simulink subsystem "Battery"  (R2022a)
settings: Solver=VariableStepAuto  StartTime=0.0  StopTime=10.0  RelTol=1e-3
settings Model: Creator=mateu  LastModifiedBy=mateu

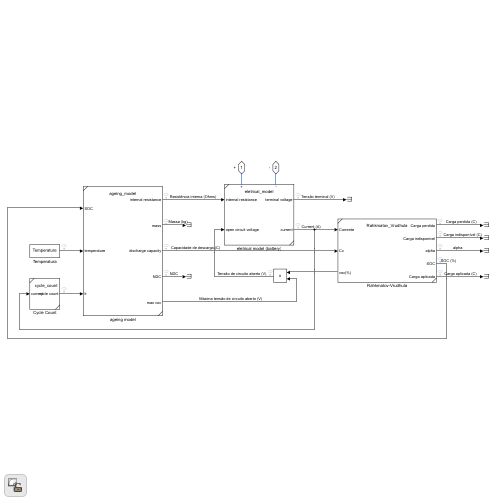
[thumbnail: Simulink's stored preview of the top-level diagram]
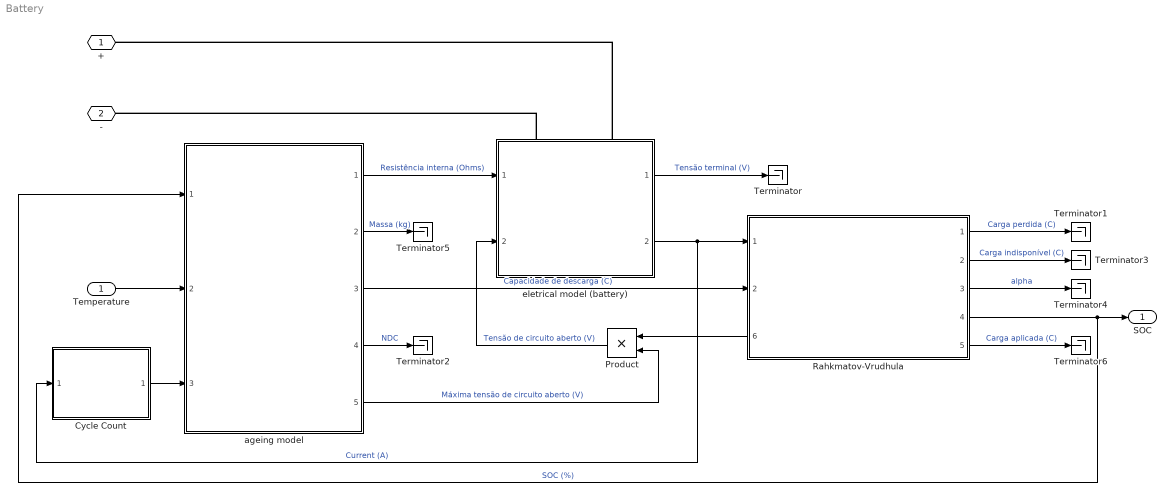
== system Battery ==
  Temperature : Inport
  Cycle Count : Subsystem  ReferencedSubsystem=cycle_count
  Product : Product
  Rahkmatov-Vrudhula : Subsystem  ReferencedSubsystem=Rahkmatov_Vrudhula
      settings: PortSchema="{\"entries\":[{\"content\":{\"sides\":[{\"content\":{\"connectorIds\":[\"In1\",\"In2\",\"Out6\"]},\"type\":\"ConnectorPlacement.EquallySpacedRectSide\",\"uuid\":\"83f3e873-db9f-47d1-b7c3-7eda48a10b32\"},{\"content\":{\"connectorIds\":[\"Out1\",\"Out2\",\"Out3\",\"Out4\",\"Out5\"],\"side\":\"RIGHT\"},\"type\":\"ConnectorPlacement.EquallySpacedRectSide\",\"uuid\":\"48ac6012-cdb4-4752-bc48-afa50bea9f0a\"},{\"content\":{\"connectorIds\":[],\"side\":\"TOP\"},\"type\":\"ConnectorPlacement.EquallySpacedRectSide\",\"uuid\":\"9cdc78bf-a718-48f1-92e6-e4070151caee\"}]},\"type\":\"ConnectorPlacement.EquallySpacedConnector\",\"uuid\":\"a231f58d-8e16-4cb4-bc80-61541bcf90eb\"}],\"packageUris\":[\"http://schema.mathworks.com/mf0/Connector/R2020b\"],\"version\":\"1.0\"}"
  Terminator{,1..6} (7 alike) : Terminator
  ageing model : Subsystem  ReferencedSubsystem=ageing_model
  eletrical model (battery) : Subsystem  ReferencedSubsystem=eletrical_model
      settings: PortSchema="{\"entries\":[{\"content\":{\"sides\":[{\"content\":{\"connectorIds\":[\"In1\",\"In2\"]},\"type\":\"ConnectorPlacement.EquallySpacedRectSide\",\"uuid\":\"e6309cc0-43d6-42db-b46d-fb5b38de698a\"},{\"content\":{\"connectorIds\":[\"Out1\",\"Out2\"],\"side\":\"RIGHT\"},\"type\":\"ConnectorPlacement.EquallySpacedRectSide\",\"uuid\":\"a3175445-87c0-47b1-a387-288225673634\"},{\"content\":{\"connectorIds\":[\"LConn2\",\"LConn1\"],\"side\":\"TOP\"},\"type\":\"ConnectorPlacement.EquallySpacedRectSide\",\"uuid\":\"f4aa44c9-f4dc-4aa8-a833-4f30710d8785\"},{\"content\":{\"connectorIds\":[],\"side\":\"BOTTOM\"},\"type\":\"ConnectorPlacement.EquallySpacedRectSide\",\"uuid\":\"f1117e0f-3189-4255-ad3f-4e2c31bb9482\"}]},\"type\":\"ConnectorPlacement.EquallySpacedConnector\",\"uuid\":\"e93a8d23-5e48-4dda-985c-f45f4ee27765\"}],\"packageUris\":[\"http://schema.mathworks.com/mf0/Connector/R2020b\"],\"version\":\"1.0\"}"
  + : PMIOPort  Side=Left
  - : PMIOPort  Port=2  Side=Left
  SOC : Outport
  wires:
  ageing model/2 -> Terminator5/1  "Massa (kg)"
  ageing model/4 -> Terminator2/1  "NDC"
  Temperature/1 -> ageing model/2
  ageing model/1 -> eletrical model (battery)/1  "Resistência interna (Ohms)"
  Cycle Count/1 -> ageing model/3
  eletrical model (battery)/2 -> Rahkmatov-Vrudhula/1, Cycle Count/1  "Current (A)"
  Rahkmatov-Vrudhula/4 -> ageing model/1, SOC/1  "SOC (%)"
  Rahkmatov-Vrudhula/3 -> Terminator4/1  "alpha"
  ageing model/5 -> Product/2  "Máxima tensão de circuito aberto (V)"
  Product/1 -> eletrical model (battery)/2  "Tensão de circuito aberto (V)"
  Rahkmatov-Vrudhula/5 -> Terminator6/1  "Carga aplicada (C)"
  eletrical model (battery)/1 -> Terminator/1  "Tensão terminal (V)"
  Rahkmatov-Vrudhula/2 -> Terminator3/1  "Carga indisponível (C)"
  Rahkmatov-Vrudhula/1 -> Terminator1/1  "Carga perdida (C)"
  Rahkmatov-Vrudhula/6 -> Product/1
  ageing model/3 -> Rahkmatov-Vrudhula/2  "Capacidade de descarga (C)"
  connections:
  eletrical model (battery)/LConn1 -- +/RConn1
  eletrical model (battery)/LConn2 -- -/RConn1
